simulink model "yawAndLaneTest_with_custom_signal"  (R2018b)
settings: Solver=FixedStepAuto  StartTime=0.0  StopTime=20  FixedStep=0.01  RelTol=1e-3
values from neighbouring files (symbols this model uses):
  ax = 0    [initialization.m]
  ay = 0    [initialization.m]
  P_init = 1    [initialization.m]
  rel_x = 0    [initialization.m]
  vx = X(2)    [cv_model_fun.m]    (also in initialization.m = 10)
  vy = X(4)    [cv_model_fun.m]    (also in initialization.m = 0)
  x = X(1)    [KinematicBicycleModel.m]    (also in SimplifiedKinematicBicycleModel.m; behavior_model.m = 0:0.01:20; cca_model_fun.m; ctra_model_fun.m)
  y = X(2)    [KinematicBicycleModel.m]    (also in SimplifiedKinematicBicycleModel.m; behavior_model.m = [distances velocities]; cca_model_fun.m; ctra_model_fun.m)
undefined symbols (not defined in the file or in its folder): sigbuilder_block
settings Model: Creator=jasprit  LastModifiedBy=jasprit

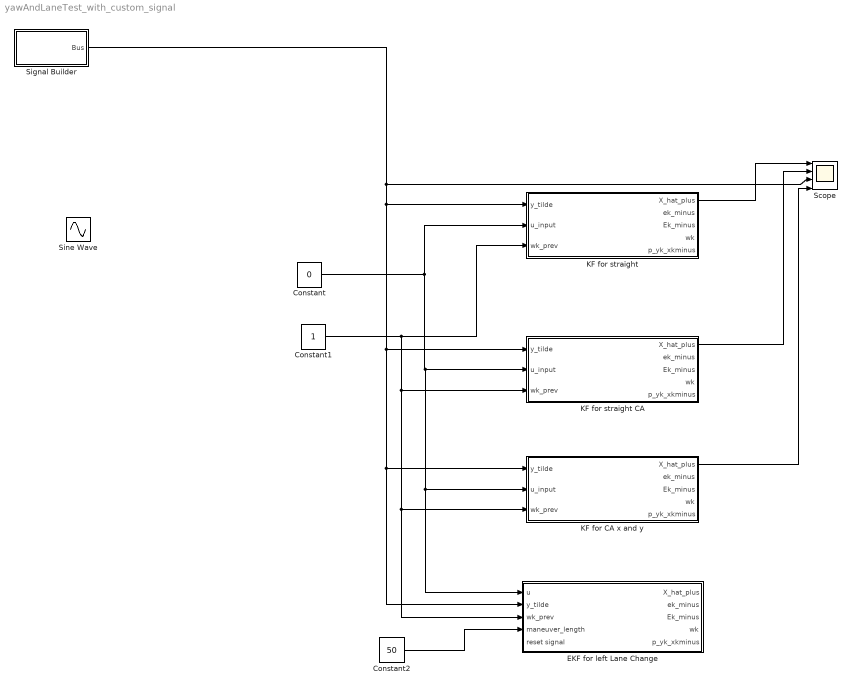
== system yawAndLaneTest_with_custom_signal ==
  Constant : Constant  Value=0
  Constant1 : Constant
  Constant2 : Constant  Value=50
  EKF for left Lane Change : Subsystem  TreatAsAtomicUnit=on
  KF for CA x and y : Subsystem
  KF for straight : Subsystem
  KF for straight CA : Subsystem
  Scope : Scope  NumInputPorts=4
  Signal Builder : Subsystem  Tag=STV Subsys  LoadFcn=sigbuilder_block('load',[545.25 0 580.5 489.75 ]);  StartFcn=sigbuilder_block('start');  StopFcn=sigbuilder_block('stop');  ClipboardFcn=sigbuilder_block('clipboard');  mask(Sigbuilder block){tuvar=[0:10]}
      mask help: Simulink:masks:SigbuilderBlock_MD
      mask init:
      | if ~strcmp(get_param(bdroot(gcbh),'SimulationStatus'),'stopped') tuvar = sigbuilder_block('maskInit'); end
      settings: CopyFcn=sigbuilder_block('copy');  DeleteFcn=sigbuilder_block('delete');  ModelCloseFcn=sigbuilder_block('modelClose');  PreSaveFcn=sigbuilder_block('preSave');  PauseFcn=sigbuilder_block('pause');  ContinueFcn=sigbuilder_block('continue');  NameChangeFcn=sigbuilder_block('namechange');  OpenFcn=sigbuilder_block('open',[549 0 573 467.25 ]);  CloseFcn=sigbuilder_block('close');
      mask Display: plot(0, 0, 100, 100,[2, 2, 32, 32, 2], [68, 8, 8, 68, 68],[32, 2], [38, 38], [32, 19, 2],[53, 60, 44], [32, 17, 17, 2],[16, 16, 31, 31]);txt = getActiveGroup(gcbh);text(2, 100, txt,'verticalAlignment', 'top');
  Sine Wave : Sin  SampleTime=0
  wires:
  Constant/1 -> EKF for left Lane Change/1(u), KF for CA x and y/2(u_input), KF for straight CA/2(u_input), KF for straight/2(u_input)
  Constant1/1 -> EKF for left Lane Change/3(wk_prev), KF for CA x and y/3(wk_prev), KF for straight CA/3(wk_prev), KF for straight/3(wk_prev)
  KF for straight/1(X_hat_plus) -> Scope/1
  KF for straight CA/1(X_hat_plus) -> Scope/2
  KF for CA x and y/1(X_hat_plus) -> Scope/4
  Signal Builder/1(Bus) -> Scope/3, EKF for left Lane Change/2(y_tilde), KF for CA x and y/1(y_tilde), KF for straight CA/1(y_tilde), KF for straight/1(y_tilde)
  Constant2/1 -> EKF for left Lane Change/4(maneuver_length)

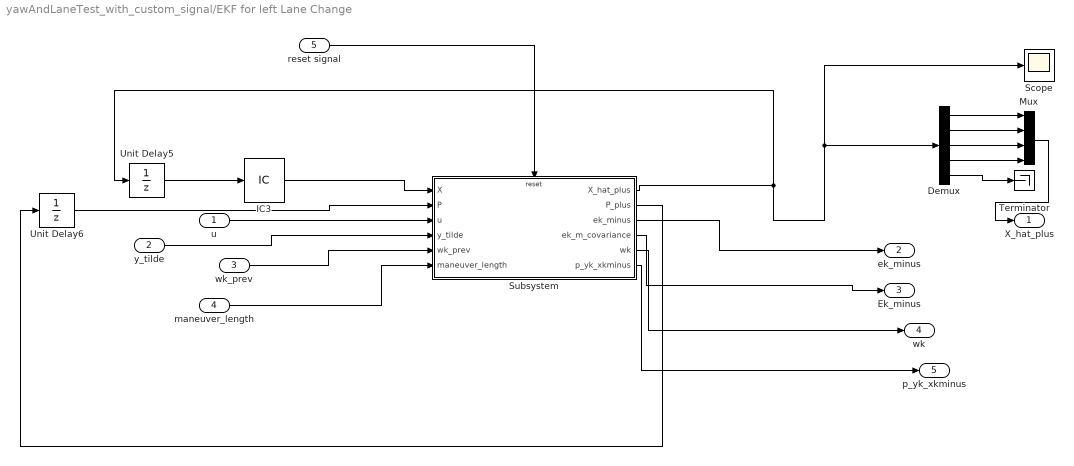
== system yawAndLaneTest_with_custom_signal/EKF for left Lane Change ==
  u : Inport
  y_tilde : Inport  Port=2
  wk_prev : Inport  Port=3
  maneuver_length : Inport  Port=4
  reset signal : Inport  Port=5
  Demux : Demux  Outputs=5
  IC3 : InitialCondition  Value=[x vx y vy rel_x]
  Mux : Mux
  Scope : Scope
  Subsystem : Subsystem
  Terminator : Terminator
  Unit Delay5 : UnitDelay  InitialCondition=[x vx y vy rel_x]  SampleTime=-1
  Unit Delay6 : UnitDelay  InitialCondition=diag([P_init, P_init, P_init, P_init, 200])  SampleTime=-1
  X_hat_plus : Outport
  ek_minus : Outport  Port=2
  Ek_minus : Outport  Port=3
  wk : Outport  Port=4
  p_yk_xkminus : Outport  Port=5
  wires:
  Mux/1 -> X_hat_plus/1
  Demux/4 -> Mux/4
  Demux/5 -> Terminator/1
  Demux/3 -> Mux/3
  Demux/2 -> Mux/2
  Unit Delay5/1 -> IC3/1
  Demux/1 -> Mux/1
  Subsystem/1(X_hat_plus) -> Demux/1, Scope/1, Unit Delay5/1
  IC3/1 -> Subsystem/1(X)
  u/1 -> Subsystem/3(u)
  y_tilde/1 -> Subsystem/4(y_tilde)
  wk_prev/1 -> Subsystem/5(wk_prev)
  maneuver_length/1 -> Subsystem/6(maneuver_length)
  Subsystem/3(ek_minus) -> ek_minus/1
  Subsystem/4(ek_m_covariance) -> Ek_minus/1
  Subsystem/5(wk) -> wk/1
  Subsystem/6(p_yk_xkminus) -> p_yk_xkminus/1
  Unit Delay6/1 -> Subsystem/2(P)
  Subsystem/2(P_plus) -> Unit Delay6/1
  reset signal/1 -> Subsystem/Reset

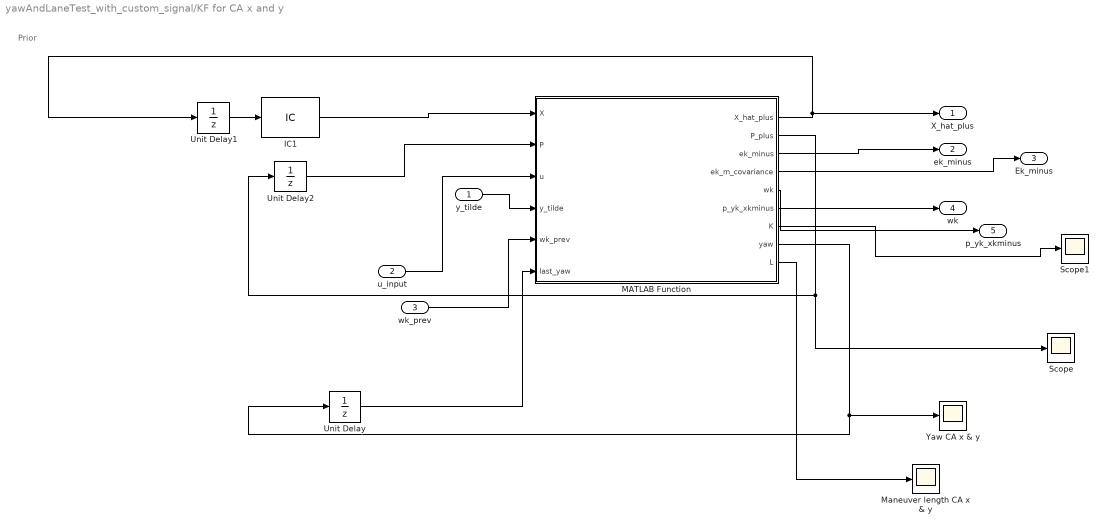
== system yawAndLaneTest_with_custom_signal/KF for CA x and y ==
  note: Prior
  y_tilde : Inport
  u_input : Inport  Port=2
  wk_prev : Inport  Port=3
  IC1 : InitialCondition  Value=[x vx ax y vy ay]
  MATLAB Function : MATLAB Function  TreatAsAtomicUnit=on
  Maneuver length CA x & y : Scope
  Scope : Scope
  Scope1 : Scope
  Unit Delay : UnitDelay  SampleTime=-1
  Unit Delay1 : UnitDelay  SampleTime=-1
  Unit Delay2 : UnitDelay  InitialCondition=eye(6)*P_init  SampleTime=-1
  Yaw CA x & y : Scope
  X_hat_plus : Outport
  ek_minus : Outport  Port=2
  Ek_minus : Outport  Port=3
  wk : Outport  Port=4
  p_yk_xkminus : Outport  Port=5
  wires:
  Unit Delay2/1 -> MATLAB Function/2(P)
  IC1/1 -> MATLAB Function/1(X)
  MATLAB Function/1(X_hat_plus) -> Unit Delay1/1, X_hat_plus/1
  u_input/1 -> MATLAB Function/3(u)
  Unit Delay1/1 -> IC1/1
  y_tilde/1 -> MATLAB Function/4(y_tilde)
  MATLAB Function/2(P_plus) -> Unit Delay2/1, Scope/1
  MATLAB Function/3(ek_minus) -> ek_minus/1
  MATLAB Function/4(ek_m_covariance) -> Ek_minus/1
  wk_prev/1 -> MATLAB Function/5(wk_prev)
  MATLAB Function/5(wk) -> wk/1
  MATLAB Function/6(p_yk_xkminus) -> p_yk_xkminus/1
  MATLAB Function/7(K) -> Scope1/1
  Unit Delay/1 -> MATLAB Function/6(last_yaw)
  MATLAB Function/8(yaw) -> Unit Delay/1, Yaw CA x & y/1
  MATLAB Function/9(L) -> Maneuver length CA x & y/1

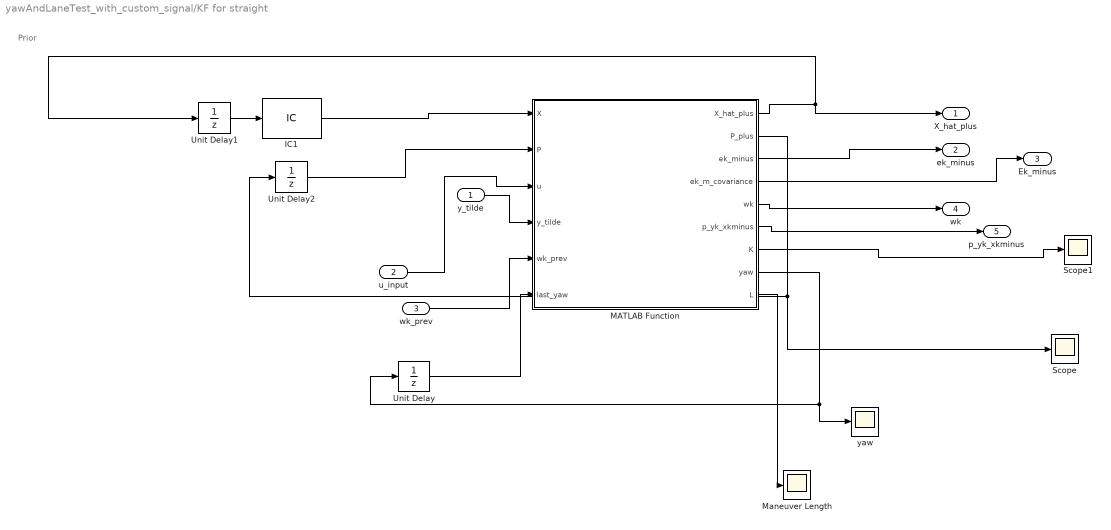
== system yawAndLaneTest_with_custom_signal/KF for straight ==
  note: Prior
  y_tilde : Inport
  u_input : Inport  Port=2
  wk_prev : Inport  Port=3
  IC1 : InitialCondition  Value=[x vx y vy]
  MATLAB Function : MATLAB Function  TreatAsAtomicUnit=on
  Maneuver Length : Scope
  Scope : Scope
  Scope1 : Scope
  Unit Delay : UnitDelay  SampleTime=-1
  Unit Delay1 : UnitDelay  SampleTime=-1
  Unit Delay2 : UnitDelay  InitialCondition=eye(4)*P_init  SampleTime=-1
  yaw : Scope
  X_hat_plus : Outport
  ek_minus : Outport  Port=2
  Ek_minus : Outport  Port=3
  wk : Outport  Port=4
  p_yk_xkminus : Outport  Port=5
  wires:
  Unit Delay2/1 -> MATLAB Function/2(P)
  IC1/1 -> MATLAB Function/1(X)
  MATLAB Function/1(X_hat_plus) -> X_hat_plus/1, Unit Delay1/1
  u_input/1 -> MATLAB Function/3(u)
  Unit Delay1/1 -> IC1/1
  y_tilde/1 -> MATLAB Function/4(y_tilde)
  MATLAB Function/2(P_plus) -> Scope/1, Unit Delay2/1
  MATLAB Function/3(ek_minus) -> ek_minus/1
  MATLAB Function/4(ek_m_covariance) -> Ek_minus/1
  wk_prev/1 -> MATLAB Function/5(wk_prev)
  MATLAB Function/5(wk) -> wk/1
  MATLAB Function/6(p_yk_xkminus) -> p_yk_xkminus/1
  MATLAB Function/7(K) -> Scope1/1
  MATLAB Function/8(yaw) -> Unit Delay/1, yaw/1
  MATLAB Function/9(L) -> Maneuver Length/1
  Unit Delay/1 -> MATLAB Function/6(last_yaw)

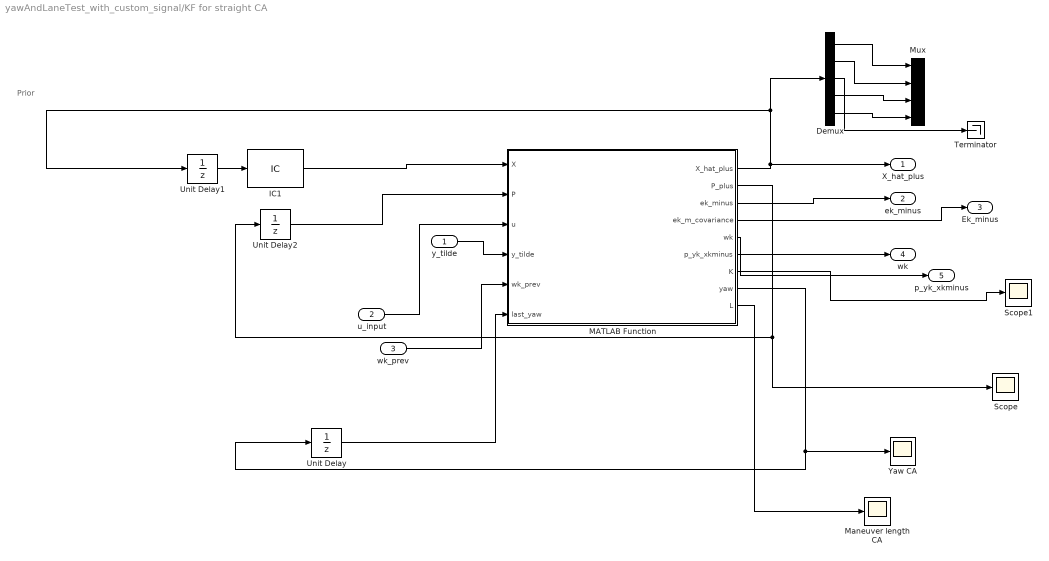
== system yawAndLaneTest_with_custom_signal/KF for straight CA ==
  note: Prior
  y_tilde : Inport
  u_input : Inport  Port=2
  wk_prev : Inport  Port=3
  Demux : Demux  Outputs=5
  IC1 : InitialCondition  Value=[x vx ax y vy]
  MATLAB Function : MATLAB Function  TreatAsAtomicUnit=on
  Maneuver length CA : Scope
  Mux : Mux
  Scope : Scope
  Scope1 : Scope
  Terminator : Terminator
  Unit Delay : UnitDelay  SampleTime=-1
  Unit Delay1 : UnitDelay  SampleTime=-1
  Unit Delay2 : UnitDelay  InitialCondition=eye(5)*P_init  SampleTime=-1
  Yaw CA : Scope
  X_hat_plus : Outport
  ek_minus : Outport  Port=2
  Ek_minus : Outport  Port=3
  wk : Outport  Port=4
  p_yk_xkminus : Outport  Port=5
  wires:
  Unit Delay2/1 -> MATLAB Function/2(P)
  IC1/1 -> MATLAB Function/1(X)
  MATLAB Function/1(X_hat_plus) -> Demux/1, Unit Delay1/1, X_hat_plus/1
  u_input/1 -> MATLAB Function/3(u)
  Unit Delay1/1 -> IC1/1
  y_tilde/1 -> MATLAB Function/4(y_tilde)
  MATLAB Function/2(P_plus) -> Unit Delay2/1, Scope/1
  MATLAB Function/3(ek_minus) -> ek_minus/1
  MATLAB Function/4(ek_m_covariance) -> Ek_minus/1
  wk_prev/1 -> MATLAB Function/5(wk_prev)
  MATLAB Function/5(wk) -> wk/1
  MATLAB Function/6(p_yk_xkminus) -> p_yk_xkminus/1
  MATLAB Function/7(K) -> Scope1/1
  Demux/1 -> Mux/1
  Demux/2 -> Mux/2
  Demux/4 -> Mux/3
  Demux/5 -> Mux/4
  Demux/3 -> Terminator/1
  Unit Delay/1 -> MATLAB Function/6(last_yaw)
  MATLAB Function/8(yaw) -> Unit Delay/1, Yaw CA/1
  MATLAB Function/9(L) -> Maneuver length CA/1

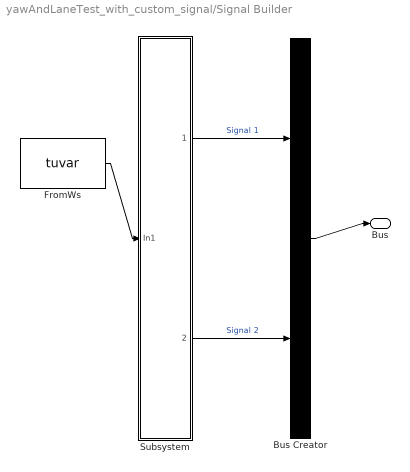
== system yawAndLaneTest_with_custom_signal/Signal Builder ==
  Bus Creator : BusCreator  Tag=Bus Creator  Inputs=2
  FromWs : FromWorkspace  Tag=STV FromWs  VariableName=tuvar  SampleTime=0
      SigBuilderData=|
      | common.afterFinalStr = 'Extrapolate'
      | common.sampleTime = 0
      | dataSet.timeRange = [0 20]
      | dataSet.name = 'Group 1'
      | sbobj.Groups.Name = 'Group 1'
      | sbobj.Groups.Signals(1).Name = 'Signal 1'
      | sbobj.Groups.Signals(1).XData = [0 0.01 0.02 0.03 0.04 0.05 0.06 0.07 0.08 0.09 0.1 0.11 ... (2001 elements, 1x2001)]
      | sbobj.Groups.Signals(1).YData = [0 0.1 0.2 0.3 0.4 0.5 0.6 0.7 0.8 0.9 1 1.1 ... (2001 elements, 1x2001)]
      | sbobj.Groups.Signals(2).Name = 'Signal 2'
      | sbobj.Groups.Signals(2).XData = [0 0.01 0.02 0.03 0.04 0.05 0.06 0.07 0.08 0.09 0.1 0.11 ... (2001 elements, 1x2001)]
      | sbobj.Groups.Signals(2).YData = [0 0 0 0 0 0 0 0 0 0 0 0 ... (2001 elements, 1x2001)]
      | sbobj.Groups.TimeRange = [0 20]
  Subsystem : Subsystem
  Bus : Outport
  wires:
  FromWs/1 -> Subsystem/1(In1)
  Bus Creator/1 -> Bus/1
  Subsystem/1(Signal 1) -> Bus Creator/1  "Signal 1"
  Subsystem/2(Signal 2) -> Bus Creator/2  "Signal 2"

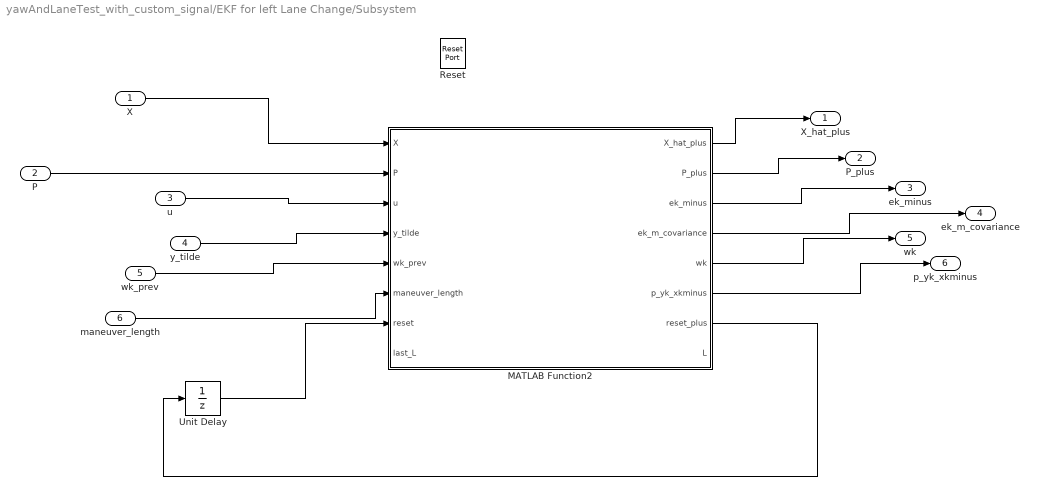
== system yawAndLaneTest_with_custom_signal/EKF for left Lane Change/Subsystem ==
  X : Inport
  P : Inport  Port=2
  u : Inport  Port=3
  y_tilde : Inport  Port=4
  wk_prev : Inport  Port=5
  maneuver_length : Inport  Port=6
  Reset : ResetPort  DisableCoverage=on
  MATLAB Function2 : MATLAB Function  TreatAsAtomicUnit=on
  Unit Delay : UnitDelay  SampleTime=-1
  X_hat_plus : Outport
  P_plus : Outport  Port=2
  ek_minus : Outport  Port=3
  ek_m_covariance : Outport  Port=4
  wk : Outport  Port=5
  p_yk_xkminus : Outport  Port=6
  wires:
  MATLAB Function2/5(wk) -> wk/1
  MATLAB Function2/1(X_hat_plus) -> X_hat_plus/1
  X/1 -> MATLAB Function2/1(X)
  P/1 -> MATLAB Function2/2(P)
  u/1 -> MATLAB Function2/3(u)
  wk_prev/1 -> MATLAB Function2/5(wk_prev)
  MATLAB Function2/3(ek_minus) -> ek_minus/1
  y_tilde/1 -> MATLAB Function2/4(y_tilde)
  maneuver_length/1 -> MATLAB Function2/6(maneuver_length)
  MATLAB Function2/2(P_plus) -> P_plus/1
  MATLAB Function2/6(p_yk_xkminus) -> p_yk_xkminus/1
  MATLAB Function2/4(ek_m_covariance) -> ek_m_covariance/1
  Unit Delay/1 -> MATLAB Function2/7(reset)
  MATLAB Function2/7(reset_plus) -> Unit Delay/1

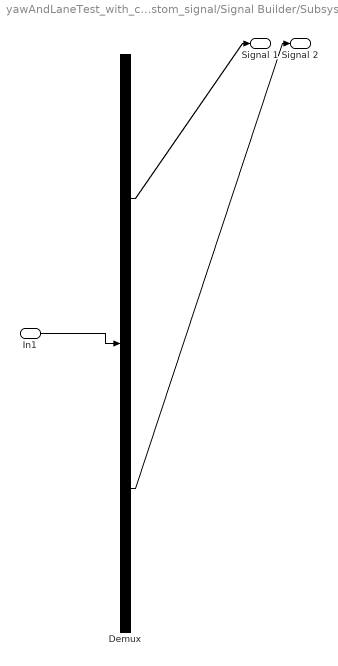
== system yawAndLaneTest_with_custom_signal/Signal Builder/Subsystem ==
  In1 : Inport
  Demux : Demux  Tag=STV Demux  Outputs=2
  Signal 1 : Outport  Tag=STV Outport
  Signal 2 : Outport  Tag=STV Outport  Port=2
  wires:
  In1/1 -> Demux/1
  Demux/1 -> Signal 1/1
  Demux/2 -> Signal 2/1

== matlab function yawAndLaneTest_with_custom_signal/KF for CA x and y/MATLAB Function ==
  data: X input; P input; u input; X_hat_plus output; y_tilde input; P_plus output; ek_minus output; ek_m_covariance output; wk output; wk_prev input; p_yk_xkminus output; K output; yaw output; L output; last_yaw input
function [X_hat_plus, P_plus, ek_minus, ek_m_covariance, wk, p_yk_xkminus, K, yaw, L] = kalmanFilterCustom(X, P, u, y_tilde, wk_prev, last_yaw)

    %%
    %TODO: See how can this be moved out of the function later
    %sampling time
    Ts_bp = 0.01;

    % measurement noise covariance
%      R = [0.25 0; 0 0.25];
   R = [0.0025 0; 0 0.0025];

       % states - X = [x vx ax y vy ay] - 

    % process noise covariance
%     Q = diag([0.5 5.0 0.5 5.0]);
%     Q = diag([0.001 0.01 0.001 0.01]);
%    Q = diag([0.01 .01 0.5 0.05 0.01]);
    a = Ts_bp^4/4;
    b = Ts_bp^3/2;
    c = Ts_bp^2;
    std_dev_q = 0.85; %m/s2
    var_q = 0.7225; %std_dev_q^2
%     Q = var_q * [a b c/2 0 0; b c Ts_bp 0 0; c/2 Ts_bp 1 0 0; 0 0 0 a b; 0 0 0 b c];
%      Q = var_q * [0.01 0 0 0 0; 0 0.01 0 0 0; 0 0 0.5 0 0; 0 0 0 var_q*a 0; 0 0 0 0 var_q*c];
    Q = diag([0.001 .001 0.001 0.001 0.001 .001]);
 

    
%     Ak = [1 Ts_bp 0 0; 0 1 0 0; 0 0 1 Ts_bp; 0 0 0 1];
    Ak = [1 Ts_bp Ts_bp^2/2 0 0 0; ...
        0 1 Ts_bp 0 0 0; ...
        0 0 1 0 0 0; ...
        0 0 0 1 Ts_bp Ts_bp^2/2; ...
        0 0 0 0 1 Ts_bp; ...
        0 0 0 0 0 1];
    Bk = 0;
    Ck = [1 0 0 0 0 0; 0 0 0 1 0 0];
    Dk = 0;

    %%
    % Now estimate states using kalman filter
    
    %predict
    xhat_minus = Ak * X + Bk * u;
%     P_minus = (Ak * P *Ak') + Ts_bp*Q;
    P_minus = (Ak * P *Ak') + Q;
    yhat_minus = Ck * xhat_minus;

    %correct
    ek_minus = y_tilde - yhat_minus;    %residual
    ek_m_covariance = Ck * P_minus *Ck' + R;    %residual covariance
    K = P_minus * Ck' * inv(ek_m_covariance);
    X_hat_plus = xhat_minus + K * ek_minus;
    P_plus = (eye(6) - K * Ck) * P_minus;
    
    %calculate MMAE weights
%     p_yk_xkminus = 1/sqrt(det(2*pi*ek_m_covariance))*exp(-1/2 * ek_minus'* inv(ek_m_covariance) * ek_minus);
    p_yk_xkminus = 1/sqrt(det((2*pi)^2*ek_m_covariance))*exp(-1/2 * ek_minus'* inv(ek_m_covariance) * ek_minus);
%     p_yk_xkminus = 1/sqrt(det((2*pi)*ek_m_covariance(2,2)))*exp(-1/2 * ek_minus(2)^2* inv(ek_m_covariance(2,2)));
    wk = wk_prev * p_yk_xkminus;
    
    %This will be likely outside
    
    %e = xhat_plus - x(:, i+1);
    
    
       % tan (yaw) = vy/vx
    yaw = atan2(X_hat_plus(5), X_hat_plus(2));
    wl = 3.5;   % lane width
    
    val = 1 - 2 * X_hat_plus(4)/wl;
    
    if val > 1
        val = 1;
    end
    
    if val < -1
        val = -1;
    end
    
    if last_yaw > 0.001    
        L = pi* wl/ (2 * tan(last_yaw))*sin(acos(val));

        if isinf(L)
            L = 0;
        end
    else
        L = 0;
    end
    
end

== matlab function yawAndLaneTest_with_custom_signal/KF for straight/MATLAB Function ==
  data: X input; P input; u input; X_hat_plus output; y_tilde input; P_plus output; ek_minus output; ek_m_covariance output; wk output; wk_prev input; p_yk_xkminus output; K output; yaw output; L output; last_yaw input
function [X_hat_plus, P_plus, ek_minus, ek_m_covariance, wk, p_yk_xkminus, K, yaw, L] = kalmanFilterCustom(X, P, u, y_tilde, wk_prev, last_yaw)

    %%
    %TODO: See how can this be moved out of the function later
    %sampling time
    Ts_bp = 0.01;

    % measurement noise covariance
%      R = [0.25 0; 0 0.25];
   R = [0.0025 0; 0 0.0025];
    
    % process noise covariance
%     Q = diag([0.5 5.0 0.5 5.0]);
    Q = diag([0.001 0.001 0.001 0.001]);

    % states - X = [x vx y vy] - 
%     X(4) = 0;
    
    Ak = [1 Ts_bp 0 0; 0 1 0 0; 0 0 1 Ts_bp; 0 0 0 1];
%     Ak = [1 Ts_bp 0 0; 0 1 0 0; 0 0 1 Ts_bp; 0 0 0 0];
    Bk = 0;
    Ck = [1 0 0 0; 0 0 1 0];
    Dk = 0;

    %%
    % Now estimate states using kalman filter
    
    %predict
    xhat_minus = Ak * X + Bk * u;
    P_minus = (Ak * P *Ak') + Ts_bp*Q;
    yhat_minus = Ck * xhat_minus;

    %correct
    ek_minus = y_tilde - yhat_minus;    %residual
    ek_m_covariance = Ck * P_minus *Ck' + R;    %residual covariance
    K = P_minus * Ck' * inv(ek_m_covariance);
    X_hat_plus = xhat_minus + K * ek_minus;
    P_plus = (eye(4) - K * Ck) * P_minus;
    
    %calculate MMAE weights
    p_yk_xkminus = 1/sqrt(det(2*pi*ek_m_covariance))*exp(-1/2 * ek_minus'* inv(ek_m_covariance) * ek_minus);
    wk = wk_prev * p_yk_xkminus;
%       wk = p_yk_xkminus;
  
    %This will be likely outside
    %e = xhat_plus - x(:, i+1);
    
    % tan (yaw) = vy/vx
    yaw = atan2(X_hat_plus(4), X_hat_plus(2));
    wl = 3.5;   % lane width
    
    val = 1 - 2 * X_hat_plus(3)/wl;
    
    if val > 1
        val = 1;
    end
    
    if val < -1
        val = -1;
    end
    
    if last_yaw > 0.001    
        L = pi* wl/ (2 * tan(last_yaw))*sin(acos(val));

        if isinf(L)
            L = 0;
        end
    else
        L = 0;
    end
    
end

== matlab function yawAndLaneTest_with_custom_signal/EKF for left Lane Change/Subsystem/MATLAB Function2 ==
  data: X input; P input; u input; X_hat_plus output; y_tilde input; P_plus output; ek_minus output; ek_m_covariance output; wk output; p_yk_xkminus output; wk_prev input; maneuver_length input; reset input; reset_plus output; last_L input; L output
function [X_hat_plus, P_plus, ek_minus, ek_m_covariance, wk, p_yk_xkminus, reset_plus, L] = EKFLeftLaneChangeCustom(X, P, u, y_tilde, wk_prev, maneuver_length, reset, last_L)

    %%
    %TODO: See how can this be moved out of the function later
    %sampling time
    Ts_bp = 0.01;
%     maneuver_length = 150;  %m
    lane_center_to_center_distance = 3.5;   %meters

    % measurement noise covariance
%      R = [0.25 0; 0 0.25];
   R = [0.0025 0; 0 0.0025];
    
    % process noise covariance
%     Q = diag([0.5 5.0 0.5 5.0]);
    Q = diag([0.001 0.001 0.001 0.001 0.001]);

    % states - X = [x vx y vy] -     
    Ck = [1 0 0 0 0 ; 0 0 1 0 0];

    if reset == 1
        reset = 0;
        
        % x0 = x, update the initiation point to x and reset the covariance
        X(5) = X(1);
        P(5,5) = 50;
    end
    
    reset_plus = reset;
    
    A = lane_center_to_center_distance/2;
    f = 1/(2*maneuver_length);
    w = 2*pi*f;
    Ts = Ts_bp;
%     F = [1 Ts 0 0 0; 0 1 0 0 0; A*w*sin(w*(x(1)-x(5))) 0 0 0 -A*w*sin(w*(x(1)-x(5))); A*w*w*x(2)*cos(w*(x(1)-x(5))) A*w*sin(w*(x(1)-x(5))) 0 0 -A*w^2*x(2)*cos(w*(x(1)-x(5))); 0 0 0 0 1];
%     F = [1 Ts 0 0 0; 0 1 0 0 0; 0 0 0 0 A*w*sin(w*x(5)); 0 A*w*sin(w*x(5)) 0 0 A*w^2*x(2)*sin(w*x(5)); 0 Ts 0 0 1];
      F = [1 Ts 0 0 0; 0 1 0 0 0; 0 0 0 0 A*w*sin(w*x(5)); 0 A*w*sin(w*x(5)) 0 0 A*w^2*x(2)*sin(w*x(5)); 0 0 0 0 1];
%     F = leftLaneChangeRelativeJacobianFcn(X, u, maneuver_length, lane_center_to_center_distance);
    %%
    % Now estimate states using kalman filter
    
    %predict
%      xhat_minus = [x(1) + x(2)*Ts_bp; x(2); -A * cos(w*(x(1)-x(5))) + A; A*w*x(2)*sin(w*(x(1)-x(5))); x(5)] + u;
    xhat_minus = [x(1) + x(2)*Ts_bp; x(2); -A * cos(w*x(5)) + A; A*w*x(2)*sin(w*x(5)); x(5)] + u;
%     xhat_minus = leftLaneChangeRelativeFcn(X, u, maneuver_length, lane_center_to_center_distance);
    P_minus = (F * P * F') + Ts_bp*Q;
    yhat_minus = Ck * xhat_minus;

    %correct
    ek_minus = y_tilde - yhat_minus;    %residual
    ek_m_covariance = Ck * P_minus *Ck' + R;    %residual covariance
    K = P_minus * Ck' * inv(ek_m_covariance);
    X_hat_plus = xhat_minus + K * ek_minus;
    P_plus = (eye(5) - K * Ck) * P_minus;
    
    %calculate MMAE weights
    p_yk_xkminus = 1/sqrt(det(2*pi*ek_m_covariance))*exp(-1/2 * ek_minus'* inv(ek_m_covariance) * ek_minus);
    wk = wk_prev * p_yk_xkminus;

    yaw = atan2(X_hat_plus(4), X_hat_plus(2));
    wl = lane_center_to_center_distance;   % lane width
    
    val = 1 - 2 * X_hat_plus(3)/wl;
    
    if val > 1
        val = 1;
    end
    
    if val < -1
        val = -1;
    end
    
    if yaw > 0.001    
        L = pi* wl/ (2 * tan(yaw))*sin(acos(val));

        if isinf(L)
            L = last_L;
        end
    else
        L = last_L;
    end
    
end

== matlab function yawAndLaneTest_with_custom_signal/KF for straight CA/MATLAB Function ==
  data: X input; P input; u input; X_hat_plus output; y_tilde input; P_plus output; ek_minus output; ek_m_covariance output; wk output; wk_prev input; p_yk_xkminus output; K output; yaw output; L output; last_yaw input
function [X_hat_plus, P_plus, ek_minus, ek_m_covariance, wk, p_yk_xkminus, K, yaw, L] = kalmanFilterCustom(X, P, u, y_tilde, wk_prev, last_yaw)

    %%
    %TODO: See how can this be moved out of the function later
    %sampling time
    Ts_bp = 0.01;

    % measurement noise covariance
%      R = [0.25 0; 0 0.25];
   R = [0.0025 0; 0 0.0025];
    
    % process noise covariance
%     Q = diag([0.5 5.0 0.5 5.0]);
%     Q = diag([0.001 0.01 0.001 0.01]);
%    Q = diag([0.01 .01 0.5 0.05 0.01]);
    a = Ts_bp^4/4;
    b = Ts_bp^3/2;
    c = Ts_bp^2;
    std_dev_q = 0.85; %m/s2
    var_q = 0.7225; %std_dev_q^2
%     Q = var_q * [a b c/2 0 0; b c Ts_bp 0 0; c/2 Ts_bp 1 0 0; 0 0 0 a b; 0 0 0 b c];
%      Q = var_q * [0.01 0 0 0 0; 0 0.01 0 0 0; 0 0 0.5 0 0; 0 0 0 var_q*a 0; 0 0 0 0 var_q*c];
    Q = diag([0.001 .001 0.001 0.001 0.001]);
 

    % states - X = [x vx y vy] - 
    
%     Ak = [1 Ts_bp 0 0; 0 1 0 0; 0 0 1 Ts_bp; 0 0 0 1];
    Ak = [1 Ts_bp Ts_bp^2/2 0 0; 0 1 Ts_bp 0 0; 0 0 1 0 0; 0 0 0 1 Ts_bp; 0 0 0 0 1];
    Bk = 0;
    Ck = [1 0 0 0 0; 0 0 0 1 0];
    Dk = 0;

    %%
    % Now estimate states using kalman filter
    
    %predict
    xhat_minus = Ak * X + Bk * u;
%     P_minus = (Ak * P *Ak') + Ts_bp*Q;
    P_minus = (Ak * P *Ak') + Q;
    yhat_minus = Ck * xhat_minus;

    %correct
    ek_minus = y_tilde - yhat_minus;    %residual
    ek_m_covariance = Ck * P_minus *Ck' + R;    %residual covariance
    K = P_minus * Ck' * inv(ek_m_covariance);
    X_hat_plus = xhat_minus + K * ek_minus;
    P_plus = (eye(5) - K * Ck) * P_minus;
    
    %calculate MMAE weights
%     p_yk_xkminus = 1/sqrt(det(2*pi*ek_m_covariance))*exp(-1/2 * ek_minus'* inv(ek_m_covariance) * ek_minus);
    p_yk_xkminus = 1/sqrt(det((2*pi)^2*ek_m_covariance))*exp(-1/2 * ek_minus'* inv(ek_m_covariance) * ek_minus);
%     p_yk_xkminus = 1/sqrt(det((2*pi)*ek_m_covariance(2,2)))*exp(-1/2 * ek_minus(2)^2* inv(ek_m_covariance(2,2)));
    wk = wk_prev * p_yk_xkminus;
    
    %This will be likely outside
    
    %e = xhat_plus - x(:, i+1);
    
    
       % tan (yaw) = vy/vx
    yaw = atan2(X_hat_plus(5), X_hat_plus(2));
    wl = 3.5;   % lane width
    
    val = 1 - 2 * X_hat_plus(4)/wl;
    
    if val > 1
        val = 1;
    end
    
    if val < -1
        val = -1;
    end
    
    if last_yaw > 0.001    
        L = pi* wl/ (2 * tan(last_yaw))*sin(acos(val));

        if isinf(L)
            L = 0;
        end
    else
        L = 0;
    end
    
end
